simulink model "boat_dynamics_model"  (R2025a)
settings: Solver=ode4  StartTime=0.0  StopTime=10  FixedStep=1e-3  RelTol=1e-3
libraries: simulink_extras x3, sim3dlib x2
settings Model: Creator=brzan  LastModifiedBy=brzan

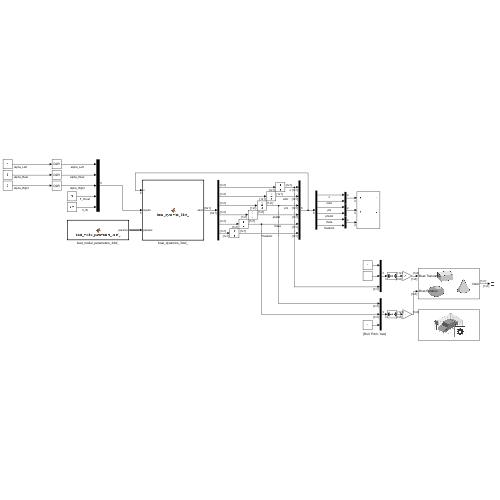
[thumbnail: Simulink's stored preview of the top-level diagram]
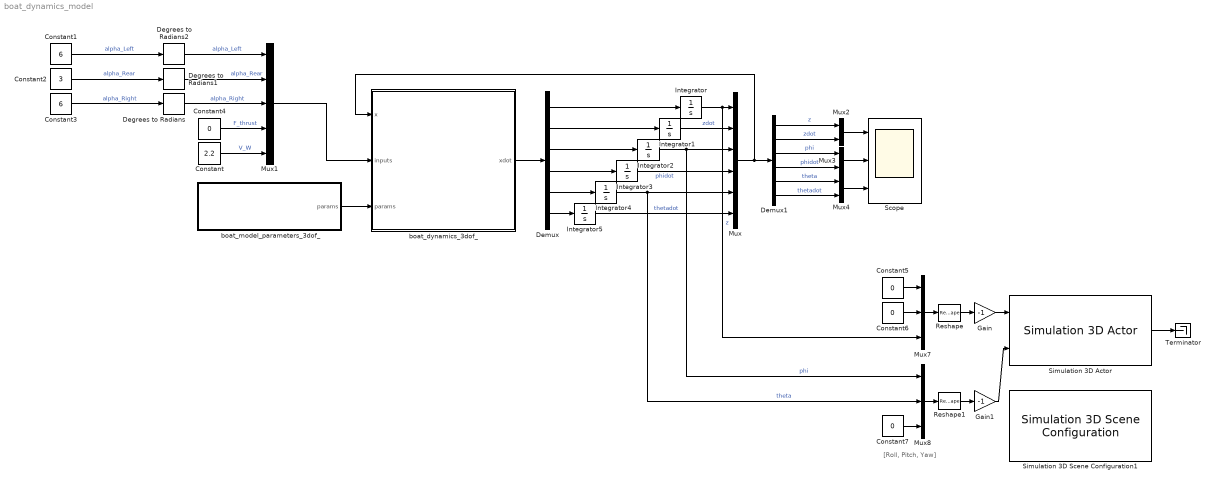
== system boat_dynamics_model ==
  note: [Roll, Pitch, Yaw]
  Constant : Constant  Value=2.2
  Constant1 : Constant  Value=6
  Constant2 : Constant  Value=3
  Constant3 : Constant  Value=6
  Constant{4..7} (4 alike) : Constant  Value=0
  Degrees to Radians : simulink_extras/Transformations/Degrees to Radians
  Degrees to Radians1 : simulink_extras/Transformations/Degrees to Radians
  Degrees to Radians2 : simulink_extras/Transformations/Degrees to Radians
  Demux : Demux  Outputs=6
  Demux1 : Demux  Outputs=6
  Gain : Gain  Gain=-1
  Gain1 : Gain  Gain=-1
  Integrator{,1..5} (6 alike) : Integrator
  Mux : Mux  Inputs=6
  Mux1 : Mux  Inputs=5
  Mux2 : Mux  Inputs=2
  Mux3 : Mux  Inputs=2
  Mux4 : Mux  Inputs=2
  Mux7 : Mux  Inputs=3
  Mux8 : Mux  Inputs=3
  Reshape : Reshape  OutputDimensionality=Row vector (2-D)
  Reshape1 : Reshape  OutputDimensionality=Row vector (2-D)
  Scope : Scope  NumInputPorts=3
      settings: ActiveDisplayYMinimum=-2.8532722674924593  ActiveDisplayYMaximum=2.75221448061251
  Simulation 3D Actor : sim3dlib/Simulation 3D Actor  Priority=1  ActorName=Boat  ParentName=Scene Origin  Operation=Create at setup  InitScriptText=|  SampleTime=-1  Translation=[0 0 0]  Rotation=[0 0 0]  Scale=[1 1 1]/1000  InputsText=Boat.Translation Boat.Rotation  aMode=5  ActorTag=Boat  ActorType=Sim3dActor  ID=C
      | % Reserved keywords:
      | % - Actor : handle to this actor object
      | % - World : handle to the world object
      | 
      | % Examples:
      | 
      | % Create a primitive geometry (optional)
      | % createShape(Actor, 'box', [1 1 1]);
      | 
      | % Initialize values (optional)
      | % Actor.Physics = true;
      | % Actor.Color = [1 0 0];
  Simulation 3D Scene Configuration1 : sim3dlib/Simulation 3D Scene Configuration  Priority=0  ProjectFormat=Default Scenes  SceneDesc=Open surface  ProjectName=C:\Program Files\MATLAB\R2025a\toolbox\shared\sim3d_projects\automotive_project_windows\UE\WindowsNoEditor\VehicleSimulation.exe  ScenePath=/Game/Maps/HwStrght  EnableOpenDRIVE=off  vehTagList={'Boat';'Custom';'Scene Origin'}  vehTag=Boat  AttachedCameraRelativeTranslation=[-4 -3 1]*1000*0.4  FreeCameraDefaultInitialTranslation=[-6, 0, 2]  AttachedCameraRelativeRotation=[0 -10 36]  FreeCameraDefaultInitialRotation=[0, -15, 0]  ViewpointName=Custom  FreeCameraInitialTranslation=[-5 0 1]  ViewpointTranslation=[0 0 0]  FreeCameraInitialRotation=[0 0 0]  ViewpointRotation=[0 0 0]  OpVisEn=off  Ts=.02  EnableWindow=on  EnableRemoteAccess=off  EnableWeather=off  SunAzimuth=90  SunAltitude=40.0  EnableGeospatialSun=off  Latitude=0  Longitude=0  Date=2023-01-01  Time=10:30:00  GeoTimeZone=-5.0  SunDaylightSaving=off  wind=1  clouds=10  EnableVolumetricClouds=off  CloudCoverage=0  CloudAltitude=6  fog=0  rain=0  RaindropsEffect=off  SnowDensity=0  EnableGeospatial=off  TilesetSource=Earth terrain  UseTrueOrigin=off  OriginHeight=200  OriginLatitude=40.744652  OriginLongitude=-73.988864  MapStyle=Aerial  AdditionalAssetIDs=[]  UseAdvancedSunSky=off  SolarTime=11  TimeZone=-5  Day=21  Month=9  Year=2022  UseDaylightSavingTime=on  DSTStartDay=10  DSTStartMonth=3  DSTEndDay=3  DSTEndMonth=11  DSTSwitchHour=2  sensorTag=MainCamera1  sensorId=1  sensorName=MainCamera1  mountLoc=Origin  offsetFlag=off  tmountOffset=[0, 0, 0]  rmountOffset=[0, 0, 0]  HorizontalResolution=1280  VerticalResolution=720  HorizontalFOV=60  mountPoint=[0 0 0]  mountOrientation=[0 0 0]  aMode=5  ID=1  GeoTrigger=Inactive  ViewNameList={'Custom'}  ViewTranslationList={'[-5 0 1]'}  ViewRotationList={'[0 0 0]'}
      settings: LibrarySourceBlock=sl3dlib/Simulation 3D/Environment/Simulation 3D Scene Configuration
  Terminator : Terminator
  boat_dynamics_3dof_ : MATLAB Function  TreatAsAtomicUnit=on
  boat_model_parameters_3dof_ : MATLAB Function  TreatAsAtomicUnit=on
  wires:
  boat_dynamics_3dof_/1(xdot) -> Demux/1
  Mux/1 -> Demux1/1, boat_dynamics_3dof_/1(x)
  boat_model_parameters_3dof_/1(params) -> boat_dynamics_3dof_/3(params)
  Demux/1 -> Integrator/1
  Demux/2 -> Integrator1/1
  Demux/4 -> Integrator3/1
  Demux/3 -> Integrator2/1
  Demux/5 -> Integrator4/1
  Demux/6 -> Integrator5/1
  Integrator/1 -> Mux7/3, Mux/1  "z"
  Integrator1/1 -> Mux/2  "zdot"
  Integrator2/1 -> Mux8/1, Mux/3  "phi"
  Integrator3/1 -> Mux/4  "phidot"
  Integrator4/1 -> Mux8/2, Mux/5  "theta"
  Integrator5/1 -> Mux/6  "thetadot"
  Constant/1 -> Mux1/5  "V_W"
  Degrees to Radians2/1 -> Mux1/1  "alpha_Left"
  Degrees to Radians1/1 -> Mux1/2  "alpha_Rear"
  Constant4/1 -> Mux1/4  "F_thrust"
  Degrees to Radians/1 -> Mux1/3  "alpha_Right"
  Mux1/1 -> boat_dynamics_3dof_/2(inputs)
  Demux1/1 -> Mux2/1  "z"
  Mux2/1 -> Scope/1
  Demux1/2 -> Mux2/2  "zdot"
  Demux1/4 -> Mux3/2  "phidot"
  Demux1/3 -> Mux3/1  "phi"
  Demux1/6 -> Mux4/2  "thetadot"
  Demux1/5 -> Mux4/1  "theta"
  Mux3/1 -> Scope/2
  Mux4/1 -> Scope/3
  Constant3/1 -> Degrees to Radians/1  "alpha_Right"
  Constant2/1 -> Degrees to Radians1/1  "alpha_Rear"
  Constant1/1 -> Degrees to Radians2/1  "alpha_Left"
  Constant5/1 -> Mux7/1
  Constant6/1 -> Mux7/2
  Mux8/1 -> Reshape1/1
  Mux7/1 -> Reshape/1
  Reshape/1 -> Gain/1
  Simulation 3D Actor/1 -> Terminator/1
  Gain1/1 -> Simulation 3D Actor/2
  Gain/1 -> Simulation 3D Actor/1
  Reshape1/1 -> Gain1/1
  Constant7/1 -> Mux8/3

== matlab function boat_dynamics_model/boat_dynamics_3dof_ ==
  data: x input; xdot output; inputs input; params input Bus: boat_model_parameters size=1
function xdot = boat_dynamics_3dof_(x, inputs, params)
%#codegen
    xdot = boat_dynamics_3dof(x, inputs, params);
end

== matlab function boat_dynamics_model/boat_model_parameters_3dof_ ==
  data: params output Bus: boat_model_parameters size=1
function params = boat_model_parameters_3dof_()
    params = boat_model_parameters_3dof();
end
